simulink model "feedback_linearization_kalman_filter_real_18_first_tun"  (R2020a)
settings: Solver=ode5  StartTime=0.0  StopTime=inf  RelTol=1e-3  EnableMultiTasking=on
undefined symbols (not defined in the file): National_Instruments, PCI, sim_output_sample_time, sim_r
libraries: sldrtlib x2, simulink x1
settings Model: Creator=wolfgang  LastModifiedBy=forale-2
settings Model: ModifiedHistory=|
  | Created an adjusted empty Simulink diagram for the lab assignments
  | in the course R0002E
settings DataIOCC: SaveFormat=Array  SignalLoggingSaveFormat=ModelDataLogs  SaveOutput=off  SignalLogging=off  DSMLogging=off  SaveTime=off  ReturnWorkspaceOutputs=off
settings OptimizationCC: ExpressionDepthLimit=2147483647  LifeSpan=inf
settings DebuggingCC: UnderspecifiedInitializationDetection=Classic  MergeDetectMultiDrivingBlocksExec=none  SolverPrmCheckMsg=warning  FcnCallInpInsideContextMsg=warning  StateNameClashWarn=warning  SFUnexpectedBacktrackingDiag=warning  SFNoUnconditionalDefaultTransitionDiag=warning  SFExecutionAtInitializationDiag=none  ArithmeticOperatorsInVariantConditions=warning
settings HardwareCC: ProdBitPerPointer=32  ProdBitPerSizeT=32  ProdBitPerPtrDiffT=32  ProdLargestAtomicFloat=None  ProdIntDivRoundTo=Undefined  ProdEndianess=Unspecified  ProdWordSize=32  ProdHWDeviceType=32-bit Generic
settings ModelReferenceCC: PropagateSignalLabelsOutOfModel=off
settings SFSimCC: SimUseLocalCustomCode=off  CustomCodeUndefinedFunction=UseInterfaceOnly
settings RTWCC: RTWUseLocalCustomCode=off
settings CodeAppCC: StateflowObjectComments=on
settings GRTTargetCC: TargetLangStandard=C89/C90 (ANSI)
settings ConfigComp: CovMetricSettings=dw  CovSaveCumulativeToWorkspaceVar=on  CovSaveSingleToWorkspaceVar=on  CovExternalEMLEnable=off  CovSFcnEnable=off

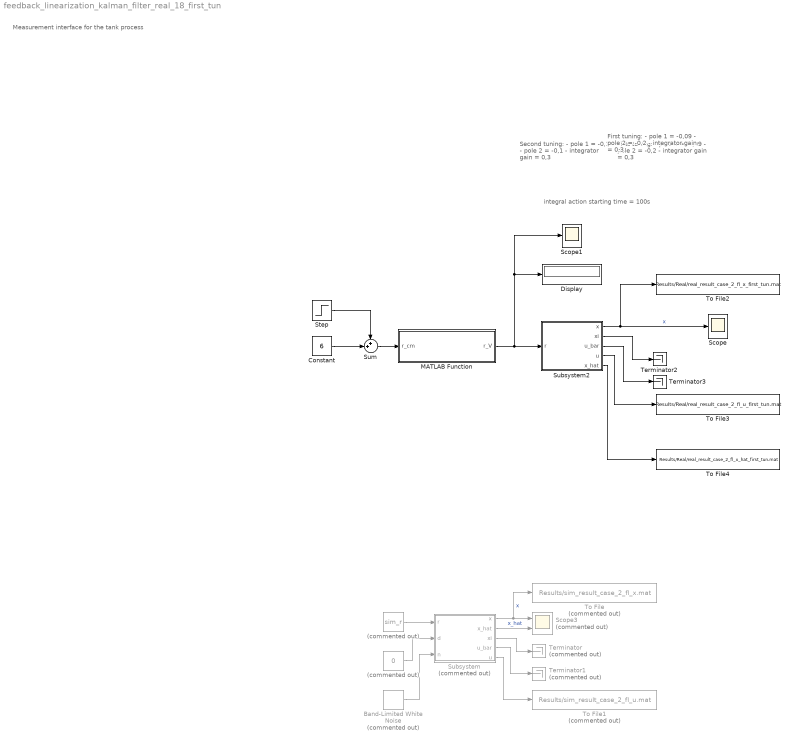
== system feedback_linearization_kalman_filter_real_18_first_tun ==
  note: integral action starting time = 100s
  note: Second tuning:
      | - pole 1 = -0,1
      | - pole 2 = -0,1
      | - integrator gain = 0,3
  note: Measurement interface for the tank process
  note: First tuning:
      | - pole 1 = -0,09
      | - pole 2 = -0,2
      | - integrator gain = 0,3
  note: First tuning:
      | - pole 1 = -0,09
      | - pole 2 = -0,2
      | - integrator gain = 0,3
  "  " : Constant  Commented=on  Value=0
  "      " : Constant  Commented=on  Value=sim_r
  Band-Limited White Noise : simulink/Sources/Band-Limited White Noise  Commented=on  Cov=0.00001  Ts=0.1  seed=[23341]
  Constant : Constant  Value=6
  Display : Display
  MATLAB Function : MATLAB Function  TreatAsAtomicUnit=on
  Scope : Scope
  Scope1 : Scope
  Scope3 : Scope  Commented=on  NumInputPorts=2
  Step : Step  Time=300  After=2  SampleTime=0
  Subsystem : Subsystem  Commented=on  mask{init_state_param=[8;8], Integrator_gain_param=0.01}
      mask prompts: init_state_param "Initial state"; Integrator_gain_param "Integrator gain"
  Subsystem2 : Subsystem  mask{pole1_param=-0.09, pole2_param=-0.2, Integrator_gain_param=0.3}
      mask prompts: pole1_param "pole1"; pole2_param "pole2"; Integrator_gain_param "Integrator gain"
  Sum : Sum  Inputs=++|
  Terminator : Terminator  Commented=on
  Terminator1 : Terminator  Commented=on
  Terminator2 : Terminator
  Terminator3 : Terminator
  To File : ToFile  Commented=on  Filename=Results/sim_result_case_2_fl_x.mat  MatrixName=sim_result_case_2_fl_x  SaveFormat=Timeseries  SampleTime=sim_output_sample_time
  To File1 : ToFile  Commented=on  Filename=Results/sim_result_case_2_fl_u.mat  MatrixName=sim_result_case_2_fl_u  SaveFormat=Timeseries  SampleTime=sim_output_sample_time
  To File2 : ToFile  Filename=Results/Real/real_result_case_2_fl_x_first_tun.mat  MatrixName=real_result_case_2_fl_x_first_tun  SaveFormat=Timeseries  SampleTime=sim_output_sample_time
  To File3 : ToFile  Filename=Results/Real/real_result_case_2_fl_u_first_tun.mat  MatrixName=real_result_case_2_fl_u_first_tun  SaveFormat=Timeseries  SampleTime=sim_output_sample_time
  To File4 : ToFile  Filename=Results/Real/real_result_case_2_fl_x_hat_first_tun.mat  MatrixName=real_result_case_2_fl_x_hat_first_tun  SaveFormat=Timeseries  SampleTime=sim_output_sample_time
  wires:
  Subsystem/2(x_hat) -> Scope3/2  "x_hat"
  "  "/1 -> Subsystem/2(d)
  "      "/1 -> Subsystem/1(r)
  Band-Limited White Noise/1 -> Subsystem/3(n)
  Subsystem/1(x) -> Scope3/1, To File/1  "x"
  Subsystem/3(xi) -> Terminator/1
  Subsystem/4(u_bar) -> Terminator1/1
  Subsystem/5(u) -> To File1/1
  Subsystem2/2(xi) -> Terminator2/1
  Subsystem2/3(u_bar) -> Terminator3/1
  Subsystem2/4(u) -> To File3/1
  Subsystem2/1(x) -> Scope/1, To File2/1  "x"
  MATLAB Function/1(r_V) -> Display/1, Scope1/1, Subsystem2/1(r)
  Constant/1 -> Sum/2
  Sum/1 -> MATLAB Function/1(r_cm)
  Step/1 -> Sum/1
  Subsystem2/5(x_hat) -> To File4/1

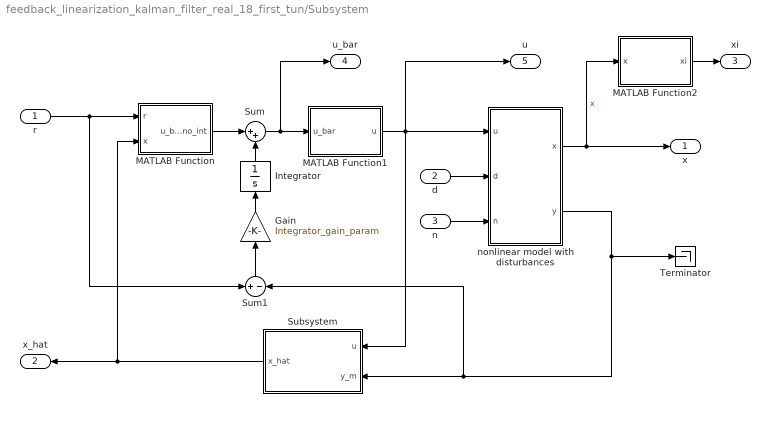
== system feedback_linearization_kalman_filter_real_18_first_tun/Subsystem ==
  r : Inport
  d : Inport  Port=2
  n : Inport  Port=3
  Gain : Gain  Gain=Integrator_gain_param
  Integrator : Integrator
  MATLAB Function : MATLAB Function  TreatAsAtomicUnit=on
  MATLAB Function1 : MATLAB Function  TreatAsAtomicUnit=on
  MATLAB Function2 : MATLAB Function  TreatAsAtomicUnit=on
  Subsystem : Subsystem
  Sum : Sum  Inputs=|++
  Sum1 : Sum  Inputs=+-
  Terminator : Terminator
  nonlinear model with disturbances : Subsystem
  x : Outport
  x_hat : Outport  Port=2
  xi : Outport  Port=3
  u_bar : Outport  Port=4
  u : Outport  Port=5
  wires:
  Sum1/1 -> Gain/1
  Gain/1 -> Integrator/1
  Integrator/1 -> Sum/2
  MATLAB Function/1(u_bar_no_int) -> Sum/1
  Sum/1 -> MATLAB Function1/1(u_bar), u_bar/1
  nonlinear model with disturbances/2(y) -> Terminator/1, Subsystem/2(y_m), Sum1/2
  MATLAB Function1/1(u) -> Subsystem/1(u), nonlinear model with disturbances/1(u), u/1
  nonlinear model with disturbances/1(x) -> MATLAB Function2/1(x), x/1  "x"
  d/1 -> nonlinear model with disturbances/2(d)
  n/1 -> nonlinear model with disturbances/3(n)
  MATLAB Function2/1(xi) -> xi/1
  r/1 -> Sum1/1, MATLAB Function/1(r)
  Subsystem/1(x_hat) -> x_hat/1, MATLAB Function/2(x)

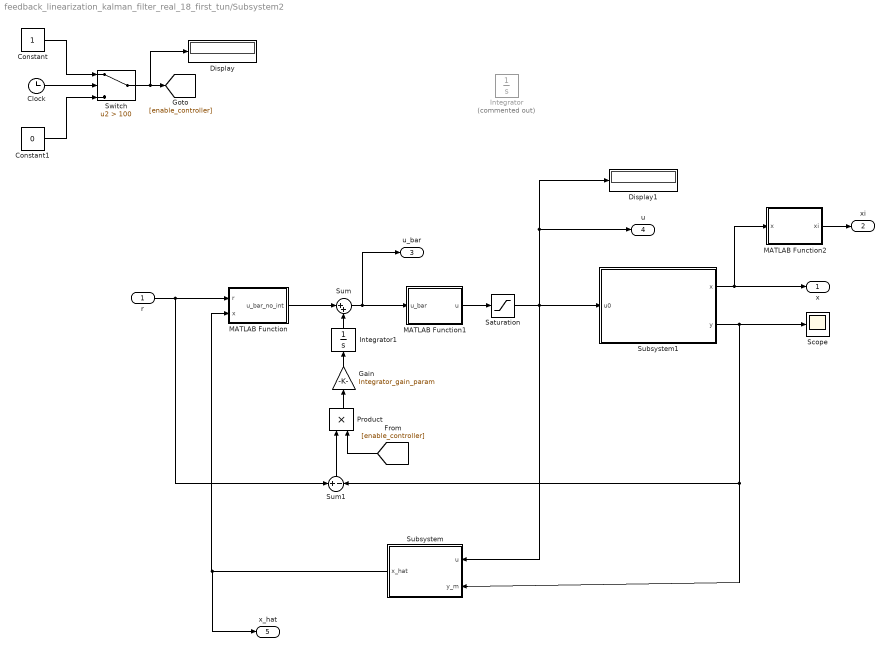
== system feedback_linearization_kalman_filter_real_18_first_tun/Subsystem2 ==
  r : Inport
  Clock : Clock
  Constant : Constant
  Constant1 : Constant  Value=0
  Display : Display
  Display1 : Display
  Gain : Gain  Gain=Integrator_gain_param
  Integrator : Integrator  Commented=on
  Integrator1 : Integrator
  MATLAB Function : MATLAB Function  TreatAsAtomicUnit=on
  MATLAB Function1 : MATLAB Function  TreatAsAtomicUnit=on
  MATLAB Function2 : MATLAB Function  TreatAsAtomicUnit=on
  Product : Product
  Saturation : Saturate  UpperLimit=10  LowerLimit=0
  Scope : Scope
  Subsystem : Subsystem
  Subsystem1 : Subsystem
  Sum : Sum  Inputs=|++
  Sum1 : Sum  Inputs=+-
  Switch : Switch  Criteria=u2 > Threshold  Threshold=100
  x : Outport
  xi : Outport  Port=2
  u_bar : Outport  Port=3
  u : Outport  Port=4
  x_hat : Outport  Port=5
  wires:
  r/1 -> MATLAB Function/1(r), Sum1/1
  MATLAB Function2/1(xi) -> xi/1
  MATLAB Function1/1(u) -> Saturation/1
  Subsystem1/1(x) -> MATLAB Function2/1(x), x/1
  Sum/1 -> u_bar/1, MATLAB Function1/1(u_bar)
  MATLAB Function/1(u_bar_no_int) -> Sum/1
  Subsystem1/2(y) -> Subsystem/2(y_m), Sum1/2, Scope/1
  Clock/1 -> Switch/2
  Constant/1 -> Switch/1
  Constant1/1 -> Switch/3
  Product/1 -> Gain/1
  Sum1/1 -> Product/1
  Switch/1 -> Display/1, [enable_controller]
  [enable_controller] -> Product/2
  Gain/1 -> Integrator1/1
  Integrator1/1 -> Sum/2
  Saturation/1 -> Subsystem/1(u), Subsystem1/1(u0), Display1/1, u/1
  Subsystem/1(x_hat) -> x_hat/1, MATLAB Function/2(x)

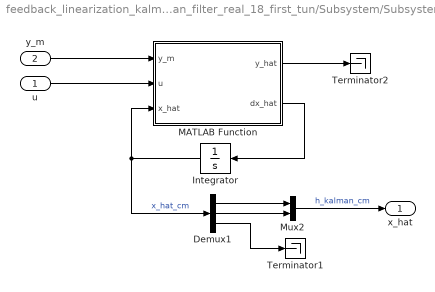
== system feedback_linearization_kalman_filter_real_18_first_tun/Subsystem/Subsystem ==
  u : Inport
  y_m : Inport  Port=2
  Demux1 : Demux  Outputs=3
  Integrator : Integrator  InitialCondition=[init_state_param;0]
  MATLAB Function : MATLAB Function  TreatAsAtomicUnit=on
  Mux2 : Mux  Inputs=2
  Terminator1 : Terminator
  Terminator2 : Terminator
  x_hat : Outport
  wires:
  Mux2/1 -> x_hat/1  "h_kalman_cm"
  MATLAB Function/2(dx_hat) -> Integrator/1
  MATLAB Function/1(y_hat) -> Terminator2/1
  y_m/1 -> MATLAB Function/1(y_m)
  u/1 -> MATLAB Function/2(u)
  Integrator/1 -> MATLAB Function/3(x_hat), Demux1/1  "x_hat_cm"
  Demux1/2 -> Mux2/2
  Demux1/1 -> Mux2/1
  Demux1/3 -> Terminator1/1

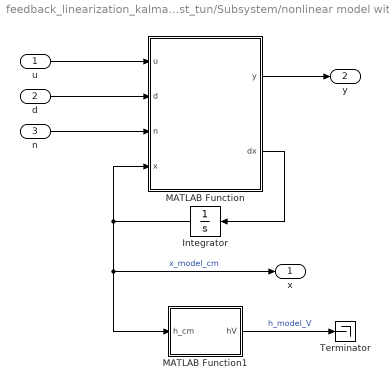
== system feedback_linearization_kalman_filter_real_18_first_tun/Subsystem/nonlinear model with disturbances ==
  u : Inport
  d : Inport  Port=2
  n : Inport  Port=3
  Integrator : Integrator  InitialCondition=init_state_param
  MATLAB Function : MATLAB Function  TreatAsAtomicUnit=on
  MATLAB Function1 : MATLAB Function  TreatAsAtomicUnit=on
  Terminator : Terminator
  x : Outport
  y : Outport  Port=2
  wires:
  u/1 -> MATLAB Function/1(u)
  Integrator/1 -> x/1, MATLAB Function1/1(h_cm), MATLAB Function/4(x)  "x_model_cm"
  MATLAB Function/2(dx) -> Integrator/1
  d/1 -> MATLAB Function/2(d)
  MATLAB Function1/1(hV) -> Terminator/1  "h_model_V"
  n/1 -> MATLAB Function/3(n)
  MATLAB Function/1(y) -> y/1

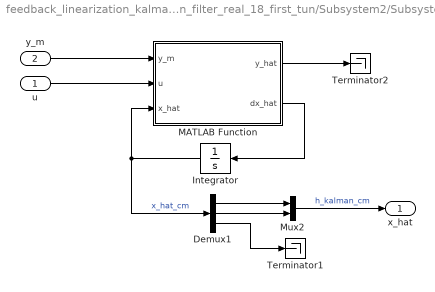
== system feedback_linearization_kalman_filter_real_18_first_tun/Subsystem2/Subsystem ==
  u : Inport
  y_m : Inport  Port=2
  Demux1 : Demux  Outputs=3
  Integrator : Integrator  InitialCondition=[0;0;0]
  MATLAB Function : MATLAB Function  TreatAsAtomicUnit=on
  Mux2 : Mux  Inputs=2
  Terminator1 : Terminator
  Terminator2 : Terminator
  x_hat : Outport
  wires:
  Mux2/1 -> x_hat/1  "h_kalman_cm"
  MATLAB Function/2(dx_hat) -> Integrator/1
  MATLAB Function/1(y_hat) -> Terminator2/1
  y_m/1 -> MATLAB Function/1(y_m)
  u/1 -> MATLAB Function/2(u)
  Integrator/1 -> MATLAB Function/3(x_hat), Demux1/1  "x_hat_cm"
  Demux1/2 -> Mux2/2
  Demux1/1 -> Mux2/1
  Demux1/3 -> Terminator1/1

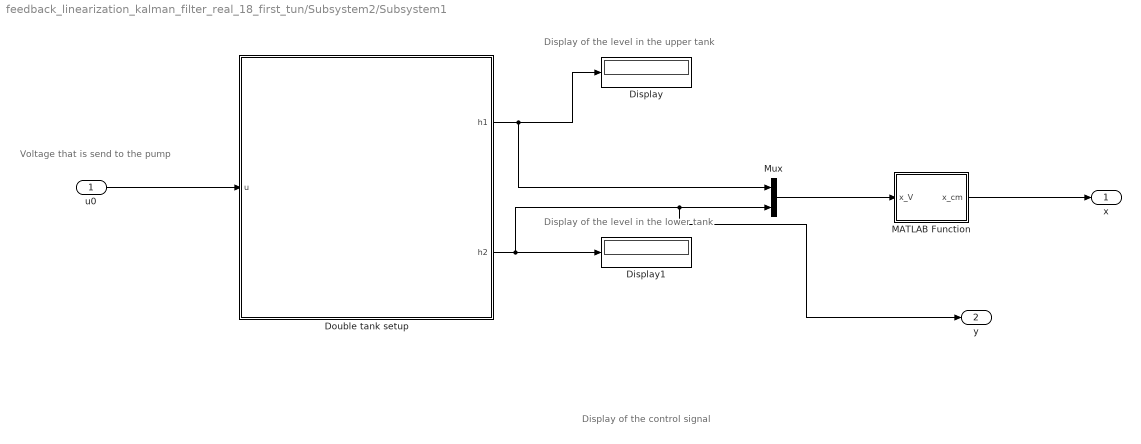
== system feedback_linearization_kalman_filter_real_18_first_tun/Subsystem2/Subsystem1 ==
  note: Voltage that is send to the pump
  note: Display of the level in the upper tank
  note: Display of the control signal
  note: Display of the level in the lower tank
  u0 : Inport
  Display : Display
  Display1 : Display
  Double tank setup : Subsystem  AncestorBlock=R0002E_lib/Double tank setup  StopFcn=|  mask(Realtime interface for the tank process){ts=0.02, h1_ch=0, h2_ch=1, u_ch=0}
      | chn =get_param(gcb,'u_ch');                          
      | s = daq.createSession('ni');                         
      | channel = ['ao',chn];                                
      | s.addAnalogOutputChannel('Dev1', channel, 'Voltage');
      | x = zeros(5,1);                                      
      | s.queueOutputData(x);                                
      | lh = s.addlistener('DataRequired', ...               
      | @(src,event) src.queueOutputData(x));                
      | s.startBackground();                                 
      | s.wait();                                            
      | s.stop();                                            
      | delete(lh);                                          
      | clear chn;                                           
      | clear s;                                             
      | clear channel;                                       
      | clear lh;                                            
      | clear x;
      mask prompts: ts "Sample time"; h1_ch "A/D Channel for upper tank"; h2_ch "A/D Channel for lower tank"; u_ch "D/A Channel for pump"
      mask help:
      | This block represents the physical interface from the computer to the tank process.
      |
      | The input u is the voltage that is provided for the pump, the output h1 is the measured level in the upper tank in [V] and the output h2 is the
      | measured level in the lower tank in [V].
      |
      | You need to provide the sample rate at which the voltage to the pump is updated and the level measurements are sampled. The sample rate should not be less than 0.02 seconds.
      mask Display:
      | x=363;
      | y=381;
      | image(imread('tank_icon.jpg'));
      | text(250/x,309/y,'Sensor');
      | text(260/x,169/y,'Sensor');
      | text(335/x,289/y,'A');
      | text(351/x,283/y,'D');
      | text(335/x,100/y,'A');
      | text(351/x,95/y,'D');
      | text(22/x,187/y,'A');
      | text(5/x,195/y,'D');
      | text(225/x,278/y,'h_1','texmode','on');
      | text(225/x,146/y,'h_2','texmode','on');
      | text(300/x,270/y,sprintf('AI-%d',h1_ch));
      | text(300/x,80/y,sprintf('AI-%d',h2_ch));
      | text(40/x,173/y,sprintf('AO-%d',u_ch));
  MATLAB Function : MATLAB Function  TreatAsAtomicUnit=on
  Mux : Mux  Inputs=2
  x : Outport
  y : Outport  Port=2
  wires:
  Double tank setup/2(h2) -> y/1, Mux/2, Display1/1
  Double tank setup/1(h1) -> Mux/1, Display/1
  u0/1 -> Double tank setup/1(u)
  MATLAB Function/1(x_cm) -> x/1
  Mux/1 -> MATLAB Function/1(x_V)

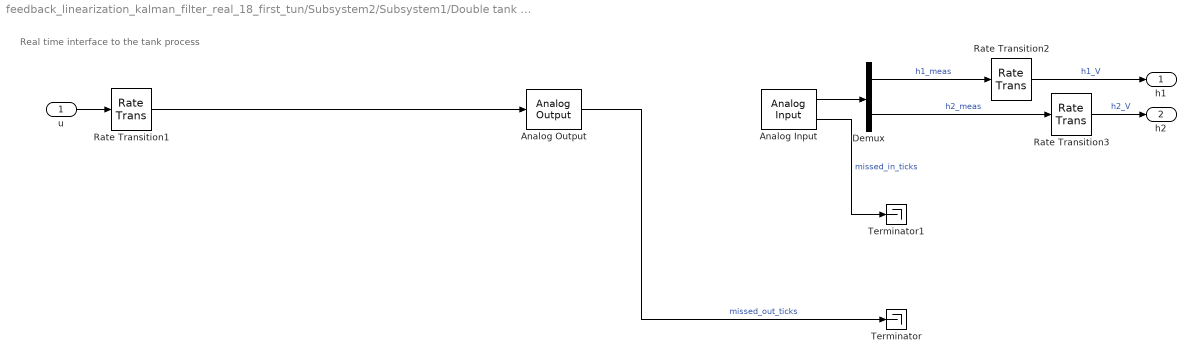
== system feedback_linearization_kalman_filter_real_18_first_tun/Subsystem2/Subsystem1/Double tank setup ==
  note: Real time interface to the tank process
  u : Inport
  Analog Input : sldrtlib/Analog Input  SampleTime=ts  MaxMissedTicks=500000000  ShowMissedTicks=on  YieldWhenWaiting=off  DrvName=National_Instruments/PCI-6024E  DrvAddress=4294967295  DrvOptions=[0 0 0 0 0 0]  Channels=[h1_ch+1,h2_ch+1]  RangeMode=1  VoltRange=1  DataType=1
      settings: AttributesFormatString=National Instruments\nPCI-6024E [auto]
  Analog Output : sldrtlib/Analog Output  SampleTime=ts  MaxMissedTicks=500000000  ShowMissedTicks=on  YieldWhenWaiting=off  DrvName=National_Instruments/PCI-6024E  DrvAddress=4294967295  DrvOptions=[0 0 0 0 0 0]  Channels=u_ch+1  RangeMode=1  VoltRange=1  InitialValue=0  FinalValue=0
      settings: AttributesFormatString=National Instruments\nPCI-6024E [auto]
  Demux : Demux  Outputs=2
  Rate Transition1 : RateTransition  OutPortSampleTime=ts
  Rate Transition2 : RateTransition
  Rate Transition3 : RateTransition
  Terminator : Terminator
  Terminator1 : Terminator
  h1 : Outport
  h2 : Outport  Port=2
  wires:
  Rate Transition1/1 -> Analog Output/1
  Rate Transition3/1 -> h2/1  "h2_V"
  Rate Transition2/1 -> h1/1  "h1_V"
  Analog Input/2 -> Terminator1/1  "missed_in_ticks"
  Demux/2 -> Rate Transition3/1  "h2_meas"
  Demux/1 -> Rate Transition2/1  "h1_meas"
  Analog Input/1 -> Demux/1
  Analog Output/1 -> Terminator/1  "missed_out_ticks"
  u/1 -> Rate Transition1/1

== matlab function feedback_linearization_kalman_filter_real_18_first_tun/Subsystem2/Subsystem/MATLAB Function ==
  data: y_hat output; y_m input; u input; x_hat input; dx_hat output
function [y_hat,dx_hat]  = kalman_filter(y_m,u,x_hat)

x1_hat = x_hat(1);
x2_hat = x_hat(2);
x3_hat = x_hat(3);

dx_hat = [x1_hat.*(-3.409145021215564e-2)-x2_hat.*4.707003693403074e-1+u.*2.098905560223644e-1+y_m.*6.312683508484582e-1-sqrt(5.0).*sqrt(7.63e+2).*x3_hat.*(4.0./5.5e+1)+9.799223895936307e-1;
    x1_hat.*3.409145021215564e-2-x2_hat.*1.823621215877479e-1+y_m.*1.98849604323964e-1+3.277173484388494e-1;x2_hat.*7.456422751238219e-3-y_m./1.0e+2-1.648066384406454e-2];

y_hat = x2_hat.*7.456422751238219e-1-1.648066384406454;

end

== matlab function feedback_linearization_kalman_filter_real_18_first_tun/Subsystem2/MATLAB Function ==
  data: r input; x input; u_bar_no_int output; pole1_param parameter; pole2_param parameter
function u_bar_no_int = k(r, x, pole1_param, pole2_param)

x1 = x(1);
x2 = x(2);
pole1 = pole1_param;
pole2 = pole2_param;

u_bar_no_int =sqrt(x1.*1.962e+3+6.2784e+3).*((pole1+pole2).*(sqrt(x1.*1.962e+3+6.2784e+3).*3.841187477910597e-3-sqrt(x2.*1.962e+3+6.2784e+3).*3.841187477910597e-3)+1.0./sqrt(x2.*1.962e+3+6.2784e+3).*(sqrt(x1.*1.962e+3+6.2784e+3).*5.151515151515152e-3-sqrt(x2.*1.962e+3+6.2784e+3).*5.151515151515152e-3).*3.768204915830296+pole1.*pole2.*r-pole1.*pole2.*(x2.*7.456422751238219e-1-1.648066384406454)+1.941196471791365e-2).*8.757485523509194;

end

== matlab function feedback_linearization_kalman_filter_real_18_first_tun/Subsystem2/Subsystem1/MATLAB Function ==
  data: x_V input; x_cm output
function x_cm = V2cm(x_V)

z = x_V;

x_cm =  1.3411256756250030495381612146841*z + 2.2102641432619661215399018079809;

end

== matlab function feedback_linearization_kalman_filter_real_18_first_tun/Subsystem/Subsystem/MATLAB Function ==
  data: y_hat output; y_m input; u input; x_hat input; dx_hat output
function [y_hat,dx_hat]  = kalman_filter(y_m,u,x_hat)

x1_hat = x_hat(1);
x2_hat = x_hat(2);
x3_hat = x_hat(3);

dx_hat = [x1_hat.*(-3.409145021215564e-2)-x2_hat.*4.707003693403074e-1+u.*2.098905560223644e-1+y_m.*6.312683508484582e-1-sqrt(5.0).*sqrt(7.63e+2).*x3_hat.*(4.0./5.5e+1)+9.799223895936307e-1;
    x1_hat.*3.409145021215564e-2-x2_hat.*1.823621215877479e-1+y_m.*1.98849604323964e-1+3.277173484388494e-1;x2_hat.*7.456422751238219e-3-y_m./1.0e+2-1.648066384406454e-2];

y_hat = x2_hat.*7.456422751238219e-1-1.648066384406454;

end

== matlab function feedback_linearization_kalman_filter_real_18_first_tun/Subsystem2/MATLAB Function1 ==
  data: u_bar input; u output
function u = pm1(u_bar)

u = u_bar.*3.277899884284337e-1-u_bar.^2.*9.88758313621772e-3+u_bar.^3.*1.567756031883916e-4-2.914041336753123;

end

== matlab function feedback_linearization_kalman_filter_real_18_first_tun/Subsystem2/MATLAB Function2 ==
  data: x input; xi output
function xi = T(x)

x1 = x(1);
x2 = x(2);

xi = [x2.*7.456422751238219e-1-1.648066384406454;sqrt(x1.*1.962e+3+6.2784e+3).*3.841187477910597e-3-sqrt(x2.*1.962e+3+6.2784e+3).*3.841187477910597e-3];

end

== matlab function feedback_linearization_kalman_filter_real_18_first_tun/Subsystem/MATLAB Function ==
  data: r input; x input; u_bar_no_int output
function u_bar_no_int = k(r,x)

x1 = x(1);
x2 = x(2);

u_bar_no_int = sqrt(x1.*1.962e+3+6.2784e+3).*(r.*(3.0./8.0e+2)-x2.*2.796158531714332e-3+1.0./sqrt(x2.*1.962e+3+6.2784e+3).*(sqrt(x1.*1.962e+3+6.2784e+3).*5.151515151515152e-3-sqrt(x2.*1.962e+3+6.2784e+3).*5.151515151515152e-3).*3.768204915830296-sqrt(x1.*1.962e+3+6.2784e+3).*4.801484347388247e-4+sqrt(x2.*1.962e+3+6.2784e+3).*4.801484347388247e-4+2.559221365943785e-2).*8.757485523509194;

end

== matlab function feedback_linearization_kalman_filter_real_18_first_tun/Subsystem/MATLAB Function1 ==
  data: u_bar input; u output
function u = pm1(u_bar)

u = u_bar.*3.277899884284337e-1-u_bar.^2.*9.88758313621772e-3+u_bar.^3.*1.567756031883916e-4-2.914041336753123;

end

== matlab function feedback_linearization_kalman_filter_real_18_first_tun/Subsystem/MATLAB Function2 ==
  data: x input; xi output
function xi = T(x)

x1 = x(1);
x2 = x(2);

xi = [x2.*7.456422751238219e-1-1.648066384406454;sqrt(x1.*1.962e+3+6.2784e+3).*3.841187477910597e-3-sqrt(x2.*1.962e+3+6.2784e+3).*3.841187477910597e-3];

end

== matlab function feedback_linearization_kalman_filter_real_18_first_tun/Subsystem/nonlinear model with disturbances/MATLAB Function ==
  data: y output; u input; dx output; d input; n input; x input
function [y,dx] = nonlinear_model(u,d,n,x)

x1 = x(1);
x2 = x(2);

y = x2.*7.456422751238219e-1 + n -1.648066384406454;

dx = [+u.*2.81859116712929e-1-(d.*sqrt(x1.*1.962e+3+6.2784e+3))./3.3e+1-sqrt(x1.*1.962e+3+6.2784e+3).*5.151515151515152e-3-u.^2.*2.476601319356692e-2+u.^3.*8.808489605974731e-4+3.751072019731428e-1;sqrt(x1.*1.962e+3+6.2784e+3).*5.151515151515152e-3-sqrt(x2.*1.962e+3+6.2784e+3).*5.151515151515152e-3];

end

== matlab function feedback_linearization_kalman_filter_real_18_first_tun/Subsystem/nonlinear model with disturbances/MATLAB Function1 ==
  data: h_cm input; hV output
function hV = g(h_cm)

hV = h_cm*7.456422751238219e-1 - 1.648066384406454;

== matlab function feedback_linearization_kalman_filter_real_18_first_tun/MATLAB Function ==
  data: r_cm input; r_V output
function r_V = i_wanna_hold_your_hand(r_cm)

z = r_cm;

r_V = 0.74564227512382186269235262443544*z - 1.6480663844064573630987524666125;

end
